simulink model "Simscape_OneUser_Modify_FK"  (R2022a)
settings: Solver=ode45  StartTime=0.0  StopTime=5  FixedStep=0.01  RelTol=1e-3
model workspace: external: MATLAB File D:\My_Data\ARAS\Eraee\0.04\Simscape_OneUser_Modify-laser_V2\Simscape_OneUser_Modify_FK_DataFile.m (data not in the file)
undefined symbols (not defined in the file or in its folder): smiData, X, Y, Z
libraries: sm_lib x164, nesl_utility x13, slpidlib x3
(part 1 of 5)
settings Model: Creator=mnaze  LastModifiedBy=mnaze

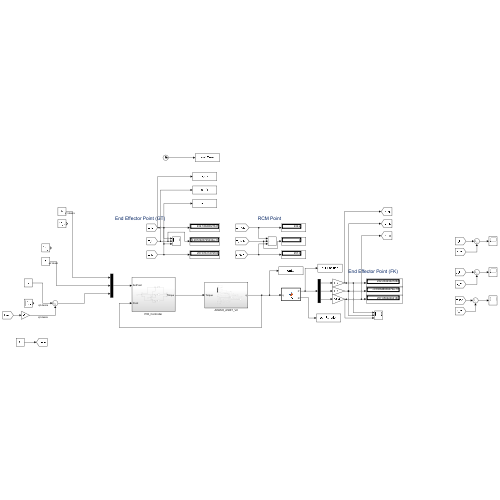
[thumbnail: Simulink's stored preview of the top-level diagram]
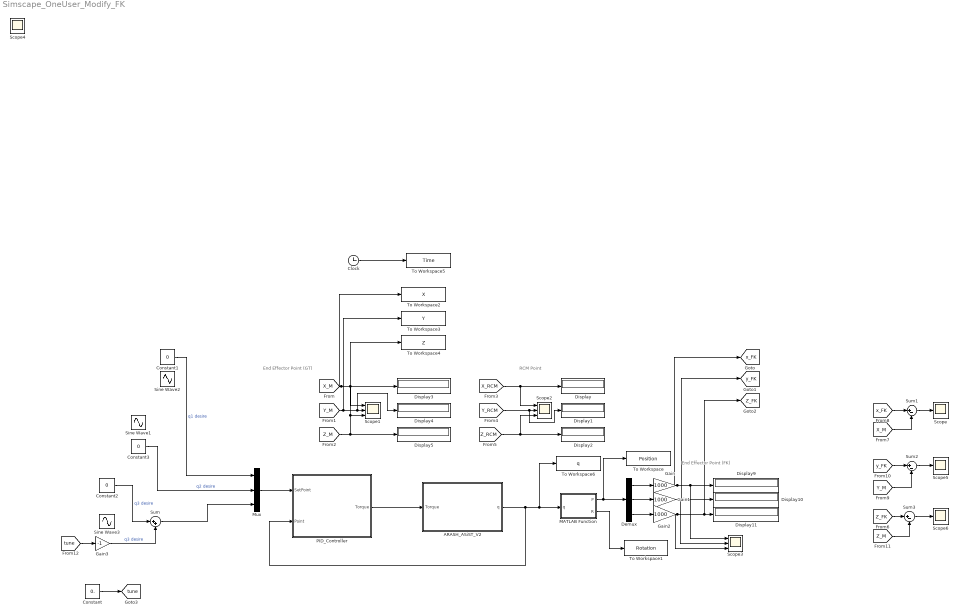
== system Simscape_OneUser_Modify_FK ==
  note: RCM Point
  note: End Effector Point (FK)
  note: End Effector Point (GT)
  ARASH_ASiST_V2 : Subsystem
  Clock : Clock
  Constant : Constant  Value=0.
  Constant1 : Constant  Value=0
  Constant2 : Constant  Value=0
  Constant3 : Constant  Value=0
  Demux : Demux  Outputs=3
  Display{,1..5,9..11} (9 alike) : Display
  Gain : Gain  Gain=1000
  Gain1 : Gain  Gain=1000
  Gain2 : Gain  Gain=1000
  Gain3 : Gain  Gain=-1
  MATLAB Function : MATLAB Function  TreatAsAtomicUnit=on
  Mux : Mux  Inputs=3
  PID_Controller : Subsystem
  Scope{,4..6} (4 alike) : Scope
  Scope1 : Scope  NumInputPorts=3
  Scope2 : Scope  NumInputPorts=3
  Scope3 : Scope  NumInputPorts=3
  Sine Wave1 : Sin  Amplitude=25  Frequency=3  SampleTime=0
  Sine Wave2 : Sin  Amplitude=45  Frequency=3  Phase=-pi/2  SampleTime=0
  Sine Wave3 : Sin  Amplitude=21  Bias=6  Frequency=3  SampleTime=0
  Sum : Sum  Inputs=|++
  Sum1 : Sum  Inputs=|+-
  Sum2 : Sum  Inputs=|+-
  Sum3 : Sum  Inputs=|+-
  To Workspace : ToWorkspace  VariableName=Position  SampleTime=-1
  To Workspace1 : ToWorkspace  VariableName=Rotation  SampleTime=-1
  To Workspace2 : ToWorkspace  VariableName=X  SampleTime=-1
  To Workspace3 : ToWorkspace  VariableName=Y  SampleTime=-1
  To Workspace4 : ToWorkspace  VariableName=Z  SampleTime=-1
  To Workspace5 : ToWorkspace  VariableName=Time  SaveFormat=Timeseries  SampleTime=-1
  To Workspace6 : ToWorkspace  VariableName=q  SampleTime=-1
  tag scope: Z_FK=global, tune=global, x_FK=global, y_FK=global
  wires:
  Constant3/1 -> Mux/2  "q2 desire"
  ARASH_ASiST_V2/1(q) -> To Workspace6/1, MATLAB Function/1(q), PID_Controller/2(Point)
  Constant1/1 -> Mux/1  "q1 desire"
  Sum/1 -> Mux/3
  Gain3/1 -> Sum/2  "q3 desire"
  PID_Controller/1(Torque) -> ARASH_ASiST_V2/1(Torque)
  MATLAB Function/1(P) -> To Workspace/1, Demux/1
  Constant2/1 -> Sum/1  "q3 desire"
  Demux/2 -> Gain1/1
  Clock/1 -> To Workspace5/1
  Gain1/1 -> Scope3/2, [y_FK], Display10/1
  Gain2/1 -> Scope3/3, [Z_FK], Display11/1
  Mux/1 -> PID_Controller/1(SetPoint)
  [Z_RCM] -> Display2/1, Scope2/3
  Demux/1 -> Gain/1
  Demux/3 -> Gain2/1
  Gain/1 -> [x_FK], Display9/1, Scope3/1
  MATLAB Function/2(R) -> To Workspace1/1
  Constant/1 -> [tune]
  [tune] -> Gain3/1
  [x_FK] -> Sum1/1
  [X_M] -> Sum1/2
  [y_FK] -> Sum2/1
  [Y_M] -> Sum2/2
  Sum2/1 -> Scope5/1
  Sum1/1 -> Scope/1
  [Z_FK] -> Sum3/1
  [Z_M] -> Sum3/2
  Sum3/1 -> Scope6/1
  [X_RCM] -> Display/1, Scope2/1
  [Y_RCM] -> Display1/1, Scope2/2
  [Z_M] -> To Workspace4/1, Scope1/3, Display5/1
  [X_M] -> Display3/1, Scope1/1, To Workspace2/1
  [Y_M] -> To Workspace3/1, Display4/1, Scope1/2
